simulink model "Tworoom_model"  (R2023a)
settings: Solver=VariableStepAuto  StartTime=0.0  StopTime=36  RelTol=1e-3
libraries: simulink x2
settings Model: Creator=oluwafemiajeigbe  LastModifiedBy=oluwafemiajeigbe

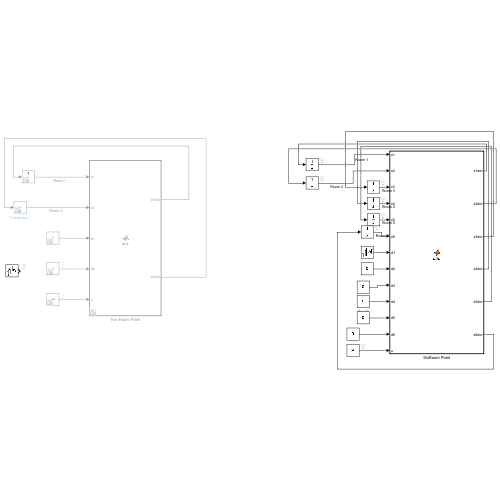
[thumbnail: Simulink's stored preview of the top-level diagram]
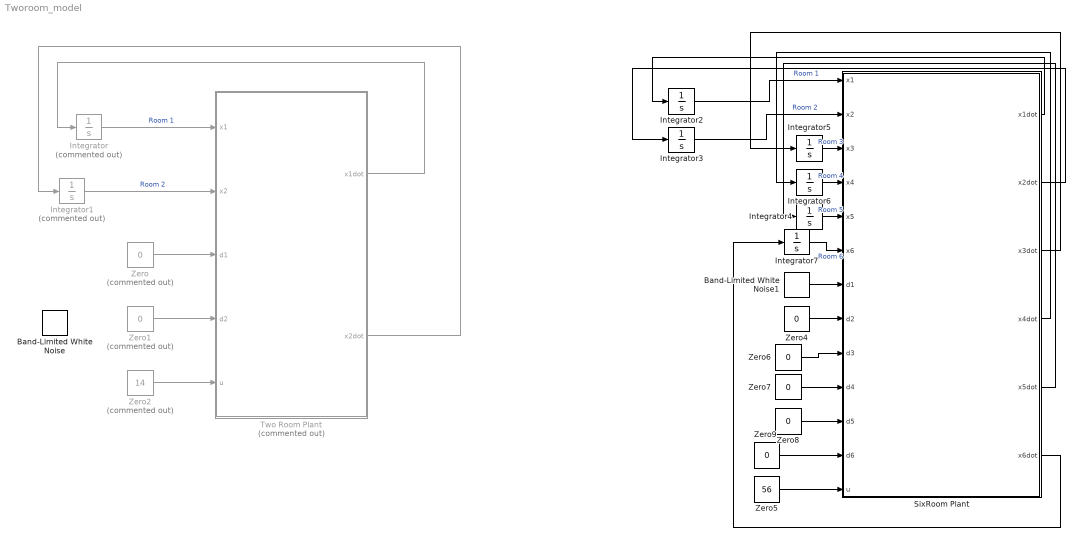
== system Tworoom_model ==
  Band-Limited White Noise : simulink/Sources/Band-Limited White Noise  Cov=[1.8]  Ts=0.1  seed=[23341]
  Band-Limited White Noise1 : simulink/Sources/Band-Limited White Noise  Cov=[18]  Ts=0.1  seed=[23341]
  Integrator : Integrator  Commented=on
  Integrator1 : Integrator  Commented=on
  Integrator{2..7} (6 alike) : Integrator
  SixRoom Plant : MATLAB Function  TreatAsAtomicUnit=on
  Two Room Plant : MATLAB Function  Commented=on  TreatAsAtomicUnit=on
  Zero : Constant  Commented=on  Value=0  OutDataTypeStr=Inherit: Inherit via back propagation
  Zero1 : Constant  Commented=on  Value=0  OutDataTypeStr=Inherit: Inherit via back propagation
  Zero2 : Constant  Commented=on  Value=14  OutDataTypeStr=Inherit: Inherit via back propagation
  Zero{4,6..9} (5 alike) : Constant  Value=0  OutDataTypeStr=Inherit: Inherit via back propagation
  Zero5 : Constant  Value=56  OutDataTypeStr=Inherit: Inherit via back propagation
  wires:
  Integrator/1 -> Two Room Plant/1(x1)  "Room 1"
  Integrator1/1 -> Two Room Plant/2(x2)  "Room 2"
  Two Room Plant/1(x1dot) -> Integrator/1
  Two Room Plant/2(x2dot) -> Integrator1/1
  Zero/1 -> Two Room Plant/3(d1)
  Zero2/1 -> Two Room Plant/5(u)
  Zero1/1 -> Two Room Plant/4(d2)
  Zero4/1 -> SixRoom Plant/8(d2)
  SixRoom Plant/1(x1dot) -> Integrator2/1
  Integrator2/1 -> SixRoom Plant/1(x1)  "Room 1"
  Integrator3/1 -> SixRoom Plant/2(x2)  "Room 2"
  SixRoom Plant/2(x2dot) -> Integrator3/1
  Zero5/1 -> SixRoom Plant/13(u)
  Integrator7/1 -> SixRoom Plant/6(x6)  "Room 6"
  Integrator5/1 -> SixRoom Plant/3(x3)  "Room 3"
  Integrator6/1 -> SixRoom Plant/4(x4)  "Room 4"
  Integrator4/1 -> SixRoom Plant/5(x5)  "Room 5"
  SixRoom Plant/5(x5dot) -> Integrator4/1
  SixRoom Plant/6(x6dot) -> Integrator7/1
  SixRoom Plant/4(x4dot) -> Integrator6/1
  SixRoom Plant/3(x3dot) -> Integrator5/1
  Zero6/1 -> SixRoom Plant/9(d3)
  Zero7/1 -> SixRoom Plant/10(d4)
  Zero8/1 -> SixRoom Plant/11(d5)
  Zero9/1 -> SixRoom Plant/12(d6)
  Band-Limited White Noise1/1 -> SixRoom Plant/7(d1)

== matlab function Tworoom_model/SixRoom Plant ==
  data: x1 input; x1dot output; x2 input; x3 input; x4 input; x5 input; x6 input; d1 input; d2 input; d3 input; d4 input; d5 input; d6 input; x2dot output; u input; x3dot output; x4dot output; x5dot output; x6dot output
function [x1dot, x2dot, x3dot, x4dot, x5dot, x6dot] = ode(x1, x2, x3, x4, x5, x6, d1, d2,  d3,  d4, d5, d6, u)

% Define Parameters
m1 = 17; % Thermal capacitance of room 1
m2 = 17; % Thermal capacitance of room 2
m3 = 17; % Thermal capacitance of room 2
m4 = 17; % Thermal capacitance of room 2
m5 = 17; % Thermal capacitance of room 2
m6 = 17; % Thermal capacitance of room 2
w12 = 0.9; % Thermal conductance between room 1 and room 2
w14 = 1.7; % Thermal conductance between room 1 and room 4
w21 = 0.8; % Thermal conductance between room 2 and room 1
w23 = 0.4; % Thermal conductance between room 2 and room 3
w25 = 1.9; % Thermal conductance between room 2 and room 5
w32 = 1.5; % Thermal conductance between room 3 and room 2
w36 = 1.4; % Thermal conductance between room 3 and room 6
w45 = 1.9; % Thermal conductance between room 4 and room 5
w54 = 1.5; % Thermal conductance between room 5 and room 4
w56 = 1.6; % Thermal conductance between room 5 and room 6
w63 = 4.3; % Thermal conductance between room 6 and room 3
w41 = 3.3; % Thermal conductance between room 6 and room 3
w52 = 3.7; % Thermal conductance between room 6 and room 3

w1o = 0.5; % Thermal conductance between room 1 and outside
w2o = 0.5; % Thermal conductance between room 2 and outside
w3o = 0.5; % Thermal conductance between room 3 and outside
w4o = 0.5; % Thermal conductance between room 4 and outside
w5o = 0.5; % Thermal conductance between room 5 and outside
w6o = 0.5; % Thermal conductance between room 6 and outside

rho = 1.2; % air density
cp = 10;  % specific heat capacity of air

gamma1 = 0.01; %fraction of the HVAC air volume to room 1
gamma2 = 0.02; %fraction of the HVAC air volume to room 2
gamma3 = 0.05; %fraction of the HVAC air volume to room 3
gamma4 = 0.10; %fraction of the HVAC air volume to room 4
gamma5 = 0.08; %fraction of the HVAC air volume to room 5
gamma6 = 0.09; %fraction of the HVAC air volume to room 6
T0 = 30; % Constant temperature of the HVAC air flow


% u=V is the control input

x1dot = 1/m1*(w21*(x2-x1) + w41*(x4-x1) - w1o*x1 + gamma1*rho*u*cp*(T0-x1)+d1);
x2dot = 1/m2*(w12*(x1-x2) +w32*(x3-x2) +w52*(x5-x2) - w2o*x2 + gamma2*rho*u*cp*(T0-x2)+d2);
x3dot = 1/m3*(w23*(x2-x3) + w63*(x6-x3) - w3o*x3 + gamma3*rho*u*cp*(T0-x3)+d3);
x4dot = 1/m4*(w14*(x1-x4) + w54*(x5-x4) - w4o*x4 + gamma4*rho*u*cp*(T0-x4)+d4);
x5dot = 1/m5*(w25*(x2-x5) + w45*(x4-x5) - w5o*x5 + gamma5*rho*u*cp*(T0-x5)+d5);
x6dot = 1/m6*(w36*(x3-x6) + w56*(x5-x6) - w6o*x6 + gamma6*rho*u*cp*(T0-x6)+d6);

== matlab function Tworoom_model/Two Room Plant ==
  data: x1 input; x1dot output; x2 input; d1 input; d2 input; x2dot output; u input
function [x1dot, x2dot] = ode(x1, x2, d1, d2, u)

%Define Parameters
m1 = 17;
m2 = 15;
w12 = 0.9;
w21 = 0.8;
w1o = 0.5;
w2o = 0.5;
rho = 1.2;
cp = 10;
gamma1 = 0.8;
gamma2 = 1.8;
T0 = 30;


% u=V is the control input
x1dot = 1/m1*(w12*(x2-x1) - w1o*x1 + gamma1*rho*u*cp*(T0-x1)+d1);
x2dot = 1/m2*(w21*(x1-x2) - w2o*x2 + gamma2*rho*u*cp*(T0-x2)+d2);
